simulink model "rw_step_test"  (R2018b)
settings: Solver=FixedStepAuto  StartTime=0.0  StopTime=60.0  FixedStep=simParams.sample_time_s  RelTol=1e-3
libraries: reaction_wheel_assembly_lib x1
settings Model: Creator=Taylor  LastModifiedBy=Taylor
settings SFSimCC: SimUseLocalCustomCode=off
settings RTWCC: RTWUseLocalCustomCode=off
settings CodeAppCC: StateflowObjectComments=on

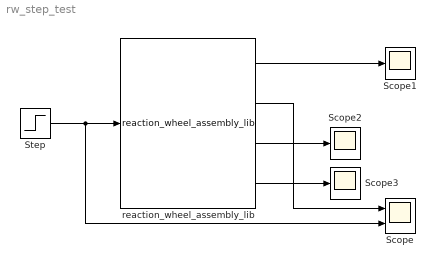
== system rw_step_test ==
  Scope : Scope  NumInputPorts=2
  Scope1 : Scope
  Scope2 : Scope
  Scope3 : Scope
  Step : Step  Time=[30 30 30 30]  Before=[1000 1000 1000 1000]  After=[1010 1010 1010 1010]  SampleTime=0
  reaction_wheel_assembly_lib : reaction_wheel_assembly_lib/reaction_wheel_assembly_lib  SystemSampleTime=-1
  wires:
  Step/1 -> reaction_wheel_assembly_lib/1, Scope/2
  reaction_wheel_assembly_lib/2 -> Scope/1
  reaction_wheel_assembly_lib/1 -> Scope1/1
  reaction_wheel_assembly_lib/3 -> Scope2/1
  reaction_wheel_assembly_lib/4 -> Scope3/1
